simulink model "closedloop_model_no_antiwindup"  (R2024a)
settings: Solver=ode45  StartTime=0.0  StopTime=10  RelTol=1e-4  AbsTol=1e-4
undefined symbols (not defined in the file): Kp, Td, Ti
libraries: cstblocks x2
settings Model: SimulationMode=accelerator  Creator=thoma  LastModifiedBy=Flo

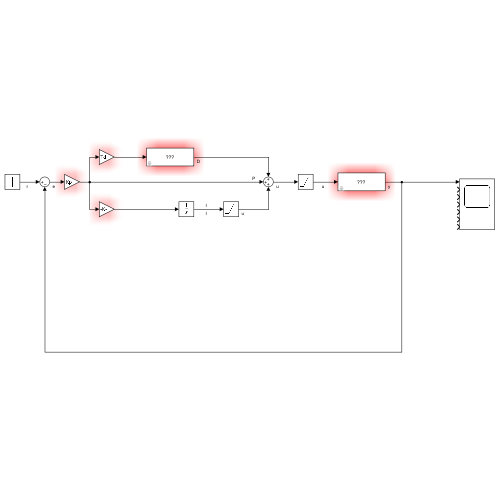
[thumbnail: Simulink's stored preview of the top-level diagram]
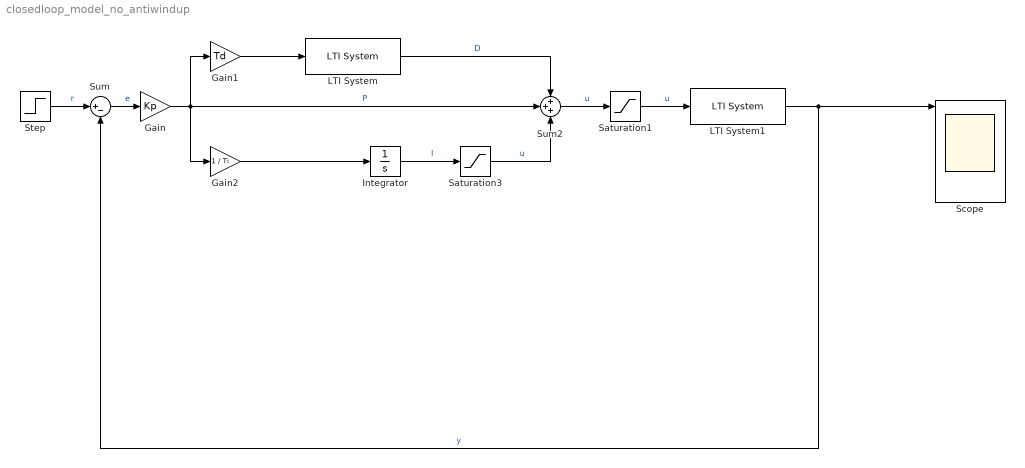
== system closedloop_model_no_antiwindup ==
  Gain : Gain  Gain=Kp
  Gain1 : Gain  Gain=Td
  Gain2 : Gain  Gain=1 / Ti
  Integrator : Integrator
  LTI System : cstblocks/LTI System  sys=F  IC=[]  PadeOrder=0
  LTI System1 : cstblocks/LTI System  sys=G  IC=[]  PadeOrder=0
  Saturation1 : Saturate  UpperLimit=5  LowerLimit=-5
  Saturation3 : Saturate  UpperLimit=5  LowerLimit=-5
  Scope : Scope  NumInputPorts=7
  Step : Step  Time=0  SampleTime=0
  Sum : Sum  Inputs=|+-
  Sum2 : Sum  Inputs=+++
  wires:
  Gain/1 -> Sum2/2, Gain1/1, Gain2/1  "P"
  Step/1 -> Sum/1  "r"
  Gain1/1 -> LTI System/1
  LTI System/1 -> Sum2/1  "D"
  LTI System1/1 -> Sum/2, Scope/1  "y"
  Sum2/1 -> Saturation1/1  "u"
  Saturation1/1 -> LTI System1/1  "u"
  Integrator/1 -> Saturation3/1  "I"
  Sum/1 -> Gain/1  "e"
  Gain2/1 -> Integrator/1
  Saturation3/1 -> Sum2/3  "u"
